simulink model "ADRC_Quanser"  (R2024a)
settings: Solver=ode1be  StartTime=0.0  StopTime=10  FixedStep=0.005  RelTol=1e-3
values from neighbouring files (symbols this model uses):
  dt = settings.dt    [Forward_Dynamics.m]    (also in Inverse_Dynamics.m; Settings.m = 0.005)
  l = settings.l    [Forward_Dynamics.m]    (also in Inverse_Dynamics.m; Settings.m = 0.127)
  omega_c = 1    [Inverse_Dynamics.m]    (also in Strojenie.m = 10^(omega_c_range(j)); Wykresy3D.m = 0.5*(omega_c_ISE + omega_c_IAE))
  P0 = [l;-l]    [Forward_Dynamics.m]    (also in Inverse_Dynamics.m)
  q0 = [0; -l/2; 3/2*pi; l/2; -l; 0; l; -l/2; pi/2; 3/2*l;0;0;-L; l;-l]    [Forward_Dynamics.m]    (also in Inverse_Dynamics.m)
libraries: slctrl_adaptive x6
settings Model: Creator=janek  LastModifiedBy=janek

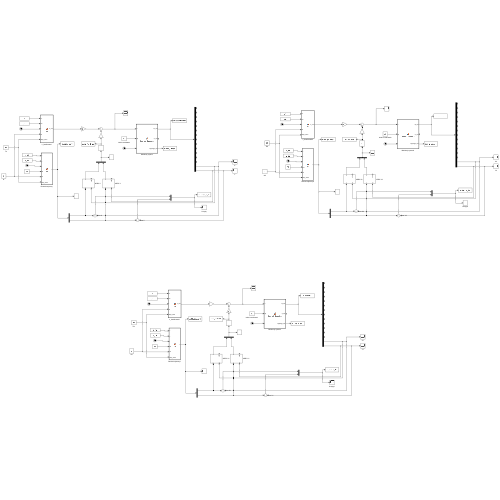
[thumbnail: Simulink's stored preview of the top-level diagram]
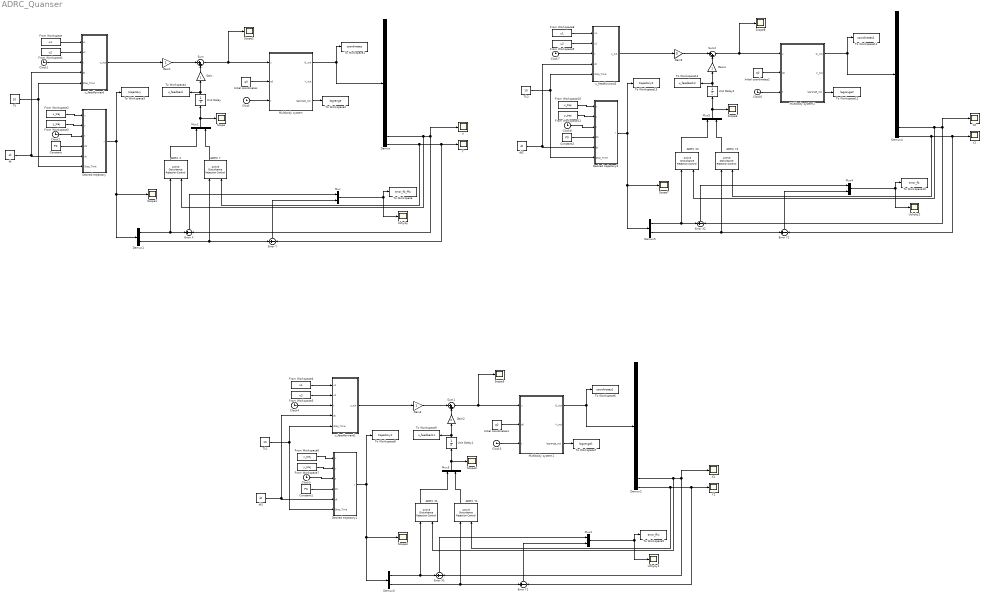
== system ADRC_Quanser ==
  ADRC X : slctrl_adaptive/Active Disturbance Rejection Control  time_domain=discrete-time  Ts=0.005  model_type=second-order  b0=b_hat  wc=omega_c*1  wo=omega_c*10  x0=[l;0;0]  ulim_checkbox=off  umax=inf  umin=-inf  xhat_checkbox=on
      settings: LibrarySourceBlock=slctrlblks/Adaptive Control/Active Disturbance Rejection Control
  ADRC X1 : slctrl_adaptive/Active Disturbance Rejection Control  time_domain=discrete-time  Ts=0.005  model_type=second-order  b0=b_hat  wc=omega_c*1  wo=omega_c*10  x0=[l;0;0]  ulim_checkbox=off  umax=inf  umin=-inf  xhat_checkbox=on
      settings: LibrarySourceBlock=slctrlblks/Adaptive Control/Active Disturbance Rejection Control
  ADRC X2 : slctrl_adaptive/Active Disturbance Rejection Control  time_domain=discrete-time  Ts=0.005  model_type=second-order  b0=b_hat  wc=omega_c*1  wo=omega_c*10  x0=[l;0;0]  ulim_checkbox=off  umax=inf  umin=-inf  xhat_checkbox=on
      settings: LibrarySourceBlock=slctrlblks/Adaptive Control/Active Disturbance Rejection Control
  ADRC Y : slctrl_adaptive/Active Disturbance Rejection Control  time_domain=discrete-time  Ts=0.005  model_type=second-order  b0=b_hat  wc=omega_c*1  wo=omega_c*10  x0=[-l;0;0]  ulim_checkbox=off  umax=inf  umin=-inf  xhat_checkbox=on
      settings: LibrarySourceBlock=slctrlblks/Adaptive Control/Active Disturbance Rejection Control
  ADRC Y1 : slctrl_adaptive/Active Disturbance Rejection Control  time_domain=discrete-time  Ts=0.005  model_type=second-order  b0=b_hat  wc=omega_c*1  wo=omega_c*10  x0=[-l;0;0]  ulim_checkbox=off  umax=inf  umin=-inf  xhat_checkbox=on
      settings: LibrarySourceBlock=slctrlblks/Adaptive Control/Active Disturbance Rejection Control
  ADRC Y2 : slctrl_adaptive/Active Disturbance Rejection Control  time_domain=discrete-time  Ts=0.005  model_type=second-order  b0=b_hat  wc=omega_c*1  wo=omega_c*10  x0=[-l;0;0]  ulim_checkbox=off  umax=inf  umin=-inf  xhat_checkbox=on
      settings: LibrarySourceBlock=slctrlblks/Adaptive Control/Active Disturbance Rejection Control
  Clock{,1..8} (9 alike) : Clock
  Constant : Constant  Value=P0
  Constant1 : Constant  Value=P0
  Constant2 : Constant  Value=P0
  Demux : Demux  Outputs=15
  Demux1 : Demux  Outputs=2
  Demux2 : Demux  Outputs=15
  Demux3 : Demux  Outputs=2
  Demux4 : Demux  Outputs=15
  Demux5 : Demux  Outputs=2
  Desired trajectory : MATLAB Function  TreatAsAtomicUnit=on
  Desired trajectory1 : MATLAB Function  TreatAsAtomicUnit=on
  Desired trajectory2 : MATLAB Function  TreatAsAtomicUnit=on
  Error X : Sum  Inputs=+|-
  Error X1 : Sum  Inputs=+|-
  Error X2 : Sum  Inputs=+|-
  Error Y : Sum  Inputs=+|-
  Error Y1 : Sum  Inputs=+|-
  Error Y2 : Sum  Inputs=+|-
  From Workspace : FromWorkspace  VariableName=u1  OutDataTypeStr=double  SampleTime=0.01
  From Workspace1 : FromWorkspace  VariableName=u2
  From Workspace10 : FromWorkspace  VariableName=x_traj
  From Workspace11 : FromWorkspace  VariableName=y_traj
  From Workspace2 : FromWorkspace  VariableName=x_traj
  From Workspace3 : FromWorkspace  VariableName=y_traj
  From Workspace4 : FromWorkspace  VariableName=u1  OutDataTypeStr=double  SampleTime=0.01
  From Workspace5 : FromWorkspace  VariableName=u2
  From Workspace6 : FromWorkspace  VariableName=x_traj
  From Workspace7 : FromWorkspace  VariableName=y_traj
  From Workspace8 : FromWorkspace  VariableName=u1  OutDataTypeStr=double  SampleTime=0.01
  From Workspace9 : FromWorkspace  VariableName=u2
  Gain{,1,3..4} (4 alike) : Gain
  Gain2 : Gain  Gain=0
  Gain5 : Gain  Gain=0
  Initial coordinates : Constant  Value=q0
  Initial coordinates1 : Constant  Value=q0
  Initial coordinates2 : Constant  Value=q0
  Multibody system : MATLAB Function  TreatAsAtomicUnit=on
  Multibody system1 : MATLAB Function  TreatAsAtomicUnit=on
  Multibody system2 : MATLAB Function  TreatAsAtomicUnit=on
  Mux{,1..5} (6 alike) : Mux  Inputs=2
  Scope{,1..8} (9 alike) : Scope
  Sum : Sum  Inputs=|++
  Sum1 : Sum  Inputs=|++
  Sum2 : Sum  Inputs=|++
  Tk : Constant  Value=10
  Tk1 : Constant  Value=10
  Tk2 : Constant  Value=10
  To Workspace : ToWorkspace  VariableName=error_fb_ffw  SaveFormat=Timeseries  SampleTime=-1
  To Workspace1 : ToWorkspace  VariableName=coordinates  SaveFormat=Timeseries  SampleTime=-1
  To Workspace10 : ToWorkspace  VariableName=error_fb  SaveFormat=Timeseries  SampleTime=-1
  To Workspace11 : ToWorkspace  VariableName=coordinates2  SaveFormat=Timeseries  SampleTime=-1
  To Workspace12 : ToWorkspace  VariableName=lagrange2  SaveFormat=Timeseries  SampleTime=-1
  To Workspace13 : ToWorkspace  VariableName=trajectory2  SaveFormat=Timeseries  SampleTime=-1
  To Workspace14 : ToWorkspace  VariableName=u_feedback2  SaveFormat=Timeseries  SampleTime=-1
  To Workspace2 : ToWorkspace  VariableName=lagrange  SaveFormat=Timeseries  SampleTime=-1
  To Workspace3 : ToWorkspace  VariableName=trajectory  SaveFormat=Timeseries  SampleTime=-1
  To Workspace4 : ToWorkspace  VariableName=u_feedback  SaveFormat=Timeseries  SampleTime=-1
  To Workspace5 : ToWorkspace  VariableName=error_ffw  SaveFormat=Timeseries  SampleTime=-1
  To Workspace6 : ToWorkspace  VariableName=coordinates1  SaveFormat=Timeseries  SampleTime=-1
  To Workspace7 : ToWorkspace  VariableName=lagrange1  SaveFormat=Timeseries  SampleTime=-1
  To Workspace8 : ToWorkspace  VariableName=trajectory1  SaveFormat=Timeseries  SampleTime=-1
  To Workspace9 : ToWorkspace  VariableName=u_feedback1  SaveFormat=Timeseries  SampleTime=-1
  Uchyby : Scope
  Uchyby1 : Scope
  Uchyby2 : Scope
  Unit Delay : UnitDelay  SampleTime=-1  HasFrameUpgradeWarning=on
  Unit Delay1 : UnitDelay  SampleTime=-1  HasFrameUpgradeWarning=on
  Unit Delay2 : UnitDelay  SampleTime=-1  HasFrameUpgradeWarning=on
  X : Scope
  X1 : Scope
  X2 : Scope
  Y : Scope
  Y1 : Scope
  Y2 : Scope
  dt : Constant  Value=dt
  dt1 : Constant  Value=dt
  dt2 : Constant  Value=dt
  u_feedforward : MATLAB Function  TreatAsAtomicUnit=on
  u_feedforward1 : MATLAB Function  TreatAsAtomicUnit=on
  u_feedforward2 : MATLAB Function  TreatAsAtomicUnit=on
  wires:
  Initial coordinates/1 -> Multibody system/2(q0)
  Multibody system/1(Q_out) -> Demux/1, To Workspace1/1
  Demux/15 -> Y/1, Error Y/2, ADRC Y/2
  Demux/14 -> ADRC X/2, X/1, Error X/2
  Multibody system/3(lagrange_out) -> To Workspace2/1
  Sum/1 -> Multibody system/1(u), Scope2/1
  Demux1/1 -> Error X/1, ADRC X/1
  Demux1/2 -> Error Y/1, ADRC Y/1
  Mux/1 -> Uchyby/1, To Workspace/1
  Clock1/1 -> u_feedforward/3(t)
  From Workspace/1 -> u_feedforward/1(u1)
  From Workspace1/1 -> u_feedforward/2(u2)
  From Workspace2/1 -> Desired trajectory/1(x)
  From Workspace3/1 -> Desired trajectory/2(y)
  Clock2/1 -> Desired trajectory/3(t)
  Desired trajectory/1(r) -> To Workspace3/1, Demux1/1, Scope1/1
  Constant/1 -> Desired trajectory/4(P0)
  Error Y/1 -> Mux/2
  Error X/1 -> Mux/1
  u_feedforward/1(u_out) -> Gain1/1
  Tk/1 -> u_feedforward/5(Stop_Time), Desired trajectory/6(Stop_Time)
  Mux1/1 -> Unit Delay/1, Scope/1
  ADRC X/1 -> Mux1/1
  ADRC Y/1 -> Mux1/2
  Unit Delay/1 -> To Workspace4/1, Gain/1
  Clock/1 -> Multibody system/3(t)
  Gain/1 -> Sum/2
  Gain1/1 -> Sum/1
  dt/1 -> u_feedforward/4(dt), Desired trajectory/5(dt)
  Constant1/1 -> Desired trajectory1/4(P0)
  Gain3/1 -> Sum1/1
  Multibody system1/3(lagrange_out) -> To Workspace7/1
  Unit Delay1/1 -> To Workspace9/1, Gain2/1
  ADRC Y1/1 -> Mux3/2
  ADRC X1/1 -> Mux3/1
  Mux3/1 -> Unit Delay1/1, Scope3/1
  Error Y1/1 -> Mux2/2
  Demux2/14 -> ADRC X1/2, X1/1, Error X1/2
  Clock5/1 -> Desired trajectory1/3(t)
  From Workspace6/1 -> Desired trajectory1/1(x)
  Demux3/1 -> Error X1/1, ADRC X1/1
  From Workspace4/1 -> u_feedforward1/1(u1)
  From Workspace7/1 -> Desired trajectory1/2(y)
  Tk1/1 -> u_feedforward1/5(Stop_Time), Desired trajectory1/6(Stop_Time)
  Clock4/1 -> u_feedforward1/3(t)
  From Workspace5/1 -> u_feedforward1/2(u2)
  Error X1/1 -> Mux2/1
  Gain2/1 -> Sum1/2
  Multibody system1/1(Q_out) -> Demux2/1, To Workspace6/1
  u_feedforward1/1(u_out) -> Gain3/1
  Clock3/1 -> Multibody system1/3(t)
  Initial coordinates1/1 -> Multibody system1/2(q0)
  dt1/1 -> u_feedforward1/4(dt), Desired trajectory1/5(dt)
  Demux2/15 -> Y1/1, Error Y1/2, ADRC Y1/2
  Mux2/1 -> Uchyby1/1, To Workspace5/1
  Demux3/2 -> Error Y1/1, ADRC Y1/1
  Sum1/1 -> Multibody system1/1(u), Scope5/1
  Desired trajectory1/1(r) -> To Workspace8/1, Demux3/1, Scope4/1
  Constant2/1 -> Desired trajectory2/4(P0)
  Gain5/1 -> Sum2/1
  Multibody system2/3(lagrange_out) -> To Workspace12/1
  Unit Delay2/1 -> To Workspace14/1, Gain4/1
  ADRC Y2/1 -> Mux5/2
  ADRC X2/1 -> Mux5/1
  Mux5/1 -> Unit Delay2/1, Scope6/1
  Error Y2/1 -> Mux4/2
  Demux4/14 -> ADRC X2/2, X2/1, Error X2/2
  Clock8/1 -> Desired trajectory2/3(t)
  From Workspace10/1 -> Desired trajectory2/1(x)
  Demux5/1 -> Error X2/1, ADRC X2/1
  From Workspace8/1 -> u_feedforward2/1(u1)
  From Workspace11/1 -> Desired trajectory2/2(y)
  Tk2/1 -> u_feedforward2/5(Stop_Time), Desired trajectory2/6(Stop_Time)
  Clock7/1 -> u_feedforward2/3(t)
  From Workspace9/1 -> u_feedforward2/2(u2)
  Error X2/1 -> Mux4/1
  Gain4/1 -> Sum2/2
  Multibody system2/1(Q_out) -> Demux4/1, To Workspace11/1
  u_feedforward2/1(u_out) -> Gain5/1
  Clock6/1 -> Multibody system2/3(t)
  Initial coordinates2/1 -> Multibody system2/2(q0)
  dt2/1 -> u_feedforward2/4(dt), Desired trajectory2/5(dt)
  Demux4/15 -> Y2/1, Error Y2/2, ADRC Y2/2
  Mux4/1 -> Uchyby2/1, To Workspace10/1
  Demux5/2 -> Error Y2/1, ADRC Y2/1
  Sum2/1 -> Multibody system2/1(u), Scope8/1
  Desired trajectory2/1(r) -> To Workspace13/1, Demux5/1, Scope7/1

== matlab function ADRC_Quanser/u_feedforward2 ==
  data: u1 input; u2 input; u_out output; t input; dt input; Stop_Time input
function u_out = fcn(u1, u2, t, dt,  Stop_Time)
if t == Stop_Time
    u_out = [0; 0];
else
u_out = [u1(round(t*1/dt) + 1); u2(round(t*1/dt) + 1)];
end

== matlab function ADRC_Quanser/Desired trajectory1 ==
  data: x input; r output; y input; t input; P0 input; dt input; Stop_Time input
function r = fcn(x, y, t,P0,dt, Stop_Time)
if t == Stop_Time   
    r = [P0(1);P0(2)];
else
    r = [x(round(t*1/dt)+1); y(round(1/dt*t)+1)];
end

== matlab function ADRC_Quanser/Desired trajectory ==
  data: x input; r output; y input; t input; P0 input; dt input; Stop_Time input
function r = fcn(x, y, t,P0,dt, Stop_Time)
if t == Stop_Time   
    r = [P0(1);P0(2)];
else
    r = [x(round(t*1/dt)+1); y(round(1/dt*t)+1)];
end

== matlab function ADRC_Quanser/Multibody system ==
  settings: updateMethod=DISCRETE
  data: u input; Q_out output; q0 input; V_out output; lagrange_out output; t input
function [Q_out, V_out, lagrange_out] = Forward_Dynamics(u, q0, t)
l = 0.127;
L = l*2;
m1 = 0.065;
m2 = 0.5*m1;
J = 9.5e-5;
g = 9.81;
M = 1.2*diag([m1,m1,J, m1,m1,J, m1,m1,J, m1,m1,J, m2,m2,m2]);

q0 = q0(1:13);
persistent initial_guess;

if isempty(initial_guess)
        % Initialize at first call
        initial_guess = [q0;l;-l; zeros(26,1)]; 
end


options = optimoptions('fsolve', 'Algorithm', 'levenberg-marquardt','FunctionTolerance', 1e-10);

func = @(unknowns)FD(unknowns, initial_guess(1:15),initial_guess(16:30),u,M,l,L,t);
solution = fsolve(func, initial_guess, options);
initial_guess = solution; % Update the guess for the next call

Q_out = solution(1:15);
V_out = solution(16:30);
lagrange_out = solution(31:end);


function solution = FD(unknowns, q, v, u, M, l, L, t)
Q = unknowns(1:15);
V = unknowns(16:30);
Lag = unknowns(31:end);

m2 = M(13,13);
g = 9.81;
dt = 0.005;



Wiatr = 0;
%WIATR
if t >= 3 && t <=3.5
    Wiatr = m2*g/100;
end

F = [0;0;u(1); 0;0;0; 0;0;0; 0;0;u(2); -m2*g;0;0];
C = Phiq(Q(1:13),Q(14:15),l);
wiezy = Phi(Q(1:13),Q(14:15),l,L);

alpha = 100;
beta = 100;

A = [M C'; C zeros(11,11)];
b = [F;Gamma(Q,V,l) - 2*alpha*C*V - beta^2*wiezy];
x = A\b;

a = x(1:15);
lagrange = x(16:end);

solution = [
V - (Q - q)/dt;
a - (V - v)/dt;
Lag - lagrange;
];

end

function jakobi = Phiq(q,p,l)
q3 = q(3);
q6 = q(6);
q9 = q(9);
q12 = q(12);
q13 = q(13);
p1 = p(1);
p2 = p(2);

jakobi=[
[-1,  0,                                                                                                                                                             -(l*sin(q3))/2,  0,  0,                                                                                                                                                                          0,  0,  0,              0,  0,  0,               0,                                                                                   0,                                                                                                                       0,                                                                                                                       0]
[ 0, -1,                                                                                                                                                              (l*cos(q3))/2,  0,  0,                                                                                                                                                                          0,  0,  0,              0,  0,  0,               0,                                                                                   0,                                                                                                                       0,                                                                                                                       0]
[ 0,  0,                                                                                                                                                                 -l*sin(q3), -1,  0,                                                                                                                                                             -(l*sin(q6))/2,  0,  0,              0,  0,  0,               0,                                                                                   0,                                                                                                                       0,                                                                                                                       0]
[ 0,  0,                                                                                                                                                                  l*cos(q3),  0, -1,                                                                                                                                                              (l*cos(q6))/2,  0,  0,              0,  0,  0,               0,                                                                                   0,                                                                                                                       0,                                                                                                                       0]
[ 0,  0,                                                                                                                                                                 -l*sin(q3),  0,  0,                                                                                                                                                                 -l*sin(q6), -1,  0, -(l*sin(q9))/2,  0,  0,               0,                                                                                   0,                                                                                                                       0,                                                                                                                       0]
[ 0,  0,                                                                                                                                                                  l*cos(q3),  0,  0,                                                                                                                                                                  l*cos(q6),  0, -1,  (l*cos(q9))/2,  0,  0,               0,                                                                                   0,                                                                                                                       0,                                                                                                                       0]
[ 0,  0,                                                                                                                                                                 -l*sin(q3),  0,  0,                                                                                                                                                                 -l*sin(q6),  0,  0,     -l*sin(q9), -1,  0, -(l*sin(q12))/2,                                                                                   0,                                                                                                                       0,                                                                                                                       0]
[ 0,  0,                                                                                                                                                                  l*cos(q3),  0,  0,                                                                                                                                                                  l*cos(q6),  0,  0,      l*cos(q9),  0, -1,  (l*cos(q12))/2,                                                                                   0,                                                                                                                       0,                                                                                                                       0]
[ 0,  0,                                                                                                                                                                 -l*sin(q3),  0,  0,                                                                                                                                                                 -l*sin(q6),  0,  0,     -l*sin(q9),  0,  0,     -l*sin(q12),                                                                                   0,                                                                                                                       0,                                                                                                                       0]
[ 0,  0,                                                                                                                                                                  l*cos(q3),  0,  0,                                                                                                                                                                  l*cos(q6),  0,  0,      l*cos(q9),  0,  0,      l*cos(q12),                                                                                   0,                                                                                                                       0,                                                                                                                       0]
[ 0,  0, -(2*l*sin(q3)*(l*cos(q3) - p1 + l*cos(q6)) - 2*l*cos(q3)*(l*sin(q3) - p2 + l*sin(q6)))/(2*((l*cos(q3) - p1 + l*cos(q6))^2 + q13^2 + (l*sin(q3) - p2 + l*sin(q6))^2)^(1/2)),  0,  0, -(2*l*sin(q6)*(l*cos(q3) - p1 + l*cos(q6)) - 2*l*cos(q6)*(l*sin(q3) - p2 + l*sin(q6)))/(2*((l*cos(q3) - p1 + l*cos(q6))^2 + q13^2 + (l*sin(q3) - p2 + l*sin(q6))^2)^(1/2)),  0,  0,              0,  0,  0,               0, q13/((l*cos(q3) - p1 + l*cos(q6))^2 + q13^2 + (l*sin(q3) - p2 + l*sin(q6))^2)^(1/2), -(2*l*cos(q3) - 2*p1 + 2*l*cos(q6))/(2*((l*cos(q3) - p1 + l*cos(q6))^2 + q13^2 + (l*sin(q3) - p2 + l*sin(q6))^2)^(1/2)), -(2*l*sin(q3) - 2*p2 + 2*l*sin(q6))/(2*((l*cos(q3) - p1 + l*cos(q6))^2 + q13^2 + (l*sin(q3) - p2 + l*sin(q6))^2)^(1/2))]
 
];
end

function wiezy = Phi(q,p,l,L)
q1 = q(1);
q2 = q(2);
q3 = q(3);
q4 = q(4);
q5 = q(5);
q6 = q(6);
q7 = q(7);
q8 = q(8);
q9 = q(9);
q10 = q(10);
q11 = q(11);
q12 = q(12);
q13 = q(13);
p1 = p(1);
p2 = p(2);

wiezy =[

 
                                                                 (l*cos(q3))/2 - q1;
                                                                 (l*sin(q3))/2 - q2;
                                                     l*cos(q3) - q4 + (l*cos(q6))/2;
                                                     l*sin(q3) - q5 + (l*sin(q6))/2;
                                         l*cos(q3) - q7 + l*cos(q6) + (l*cos(q9))/2;
                                         l*sin(q3) - q8 + l*sin(q6) + (l*sin(q9))/2;
                           l*cos(q3) - q10 + l*cos(q6) + l*cos(q9) + (l*cos(q12))/2;
                           l*sin(q3) - q11 + l*sin(q6) + l*sin(q9) + (l*sin(q12))/2;
                               l*cos(q3) - 2*l + l*cos(q6) + l*cos(q9) + l*cos(q12);
                                     l*sin(q3) + l*sin(q6) + l*sin(q9) + l*sin(q12);
((l*cos(q3) - p1 + l*cos(q6))^2 + q13^2 + (l*sin(q3) - p2 + l*sin(q6))^2)^(1/2) - L;
];
 
                                                                
end

end

== matlab function ADRC_Quanser/u_feedforward ==
  data: u1 input; u2 input; u_out output; t input; dt input; Stop_Time input
function u_out = fcn(u1, u2, t, dt,  Stop_Time)
if t == Stop_Time
    u_out = [0; 0];
else
u_out = [u1(round(t*1/dt) + 1); u2(round(t*1/dt) + 1)];
end

== matlab function ADRC_Quanser/Multibody system1 ==
  settings: updateMethod=DISCRETE
  data: u input; Q_out output; q0 input; V_out output; lagrange_out output; t input
function [Q_out, V_out, lagrange_out] = Forward_Dynamics(u, q0, t)
l = 0.127;
L = l*2;
m1 = 0.065;
m2 = 0.5*m1;
J = 9.5e-5;
g = 9.81;
M = 1.2*diag([m1,m1,J, m1,m1,J, m1,m1,J, m1,m1,J, m2,m2,m2]);

q0 = q0(1:13);
persistent initial_guess;

if isempty(initial_guess)
        % Initialize at first call
        initial_guess = [q0;l;-l; zeros(26,1)]; 
end


options = optimoptions('fsolve', 'Algorithm', 'levenberg-marquardt','FunctionTolerance', 1e-10);

func = @(unknowns)FD(unknowns, initial_guess(1:15),initial_guess(16:30),u,M,l,L,t);
solution = fsolve(func, initial_guess, options);
initial_guess = solution; % Update the guess for the next call

Q_out = solution(1:15);
V_out = solution(16:30);
lagrange_out = solution(31:end);


function solution = FD(unknowns, q, v, u, M, l, L, t)
Q = unknowns(1:15);
V = unknowns(16:30);
Lag = unknowns(31:end);

m2 = M(13,13);
g = 9.81;
dt = 0.005;



Wiatr = 0;
%WIATR
if t >= 3 && t <=3.5
    Wiatr = m2*g/100;
end

F = [0;0;u(1); 0;0;0; 0;0;0; 0;0;u(2); -m2*g;0;0];
C = Phiq(Q(1:13),Q(14:15),l);
wiezy = Phi(Q(1:13),Q(14:15),l,L);

alpha = 100;
beta = 100;

A = [M C'; C zeros(11,11)];
b = [F;Gamma(Q,V,l) - 2*alpha*C*V - beta^2*wiezy];
x = A\b;

a = x(1:15);
lagrange = x(16:end);

solution = [
V - (Q - q)/dt;
a - (V - v)/dt;
Lag - lagrange;
];

end

function jakobi = Phiq(q,p,l)
q3 = q(3);
q6 = q(6);
q9 = q(9);
q12 = q(12);
q13 = q(13);
p1 = p(1);
p2 = p(2);

jakobi=[
[-1,  0,                                                                                                                                                             -(l*sin(q3))/2,  0,  0,                                                                                                                                                                          0,  0,  0,              0,  0,  0,               0,                                                                                   0,                                                                                                                       0,                                                                                                                       0]
[ 0, -1,                                                                                                                                                              (l*cos(q3))/2,  0,  0,                                                                                                                                                                          0,  0,  0,              0,  0,  0,               0,                                                                                   0,                                                                                                                       0,                                                                                                                       0]
[ 0,  0,                                                                                                                                                                 -l*sin(q3), -1,  0,                                                                                                                                                             -(l*sin(q6))/2,  0,  0,              0,  0,  0,               0,                                                                                   0,                                                                                                                       0,                                                                                                                       0]
[ 0,  0,                                                                                                                                                                  l*cos(q3),  0, -1,                                                                                                                                                              (l*cos(q6))/2,  0,  0,              0,  0,  0,               0,                                                                                   0,                                                                                                                       0,                                                                                                                       0]
[ 0,  0,                                                                                                                                                                 -l*sin(q3),  0,  0,                                                                                                                                                                 -l*sin(q6), -1,  0, -(l*sin(q9))/2,  0,  0,               0,                                                                                   0,                                                                                                                       0,                                                                                                                       0]
[ 0,  0,                                                                                                                                                                  l*cos(q3),  0,  0,                                                                                                                                                                  l*cos(q6),  0, -1,  (l*cos(q9))/2,  0,  0,               0,                                                                                   0,                                                                                                                       0,                                                                                                                       0]
[ 0,  0,                                                                                                                                                                 -l*sin(q3),  0,  0,                                                                                                                                                                 -l*sin(q6),  0,  0,     -l*sin(q9), -1,  0, -(l*sin(q12))/2,                                                                                   0,                                                                                                                       0,                                                                                                                       0]
[ 0,  0,                                                                                                                                                                  l*cos(q3),  0,  0,                                                                                                                                                                  l*cos(q6),  0,  0,      l*cos(q9),  0, -1,  (l*cos(q12))/2,                                                                                   0,                                                                                                                       0,                                                                                                                       0]
[ 0,  0,                                                                                                                                                                 -l*sin(q3),  0,  0,                                                                                                                                                                 -l*sin(q6),  0,  0,     -l*sin(q9),  0,  0,     -l*sin(q12),                                                                                   0,                                                                                                                       0,                                                                                                                       0]
[ 0,  0,                                                                                                                                                                  l*cos(q3),  0,  0,                                                                                                                                                                  l*cos(q6),  0,  0,      l*cos(q9),  0,  0,      l*cos(q12),                                                                                   0,                                                                                                                       0,                                                                                                                       0]
[ 0,  0, -(2*l*sin(q3)*(l*cos(q3) - p1 + l*cos(q6)) - 2*l*cos(q3)*(l*sin(q3) - p2 + l*sin(q6)))/(2*((l*cos(q3) - p1 + l*cos(q6))^2 + q13^2 + (l*sin(q3) - p2 + l*sin(q6))^2)^(1/2)),  0,  0, -(2*l*sin(q6)*(l*cos(q3) - p1 + l*cos(q6)) - 2*l*cos(q6)*(l*sin(q3) - p2 + l*sin(q6)))/(2*((l*cos(q3) - p1 + l*cos(q6))^2 + q13^2 + (l*sin(q3) - p2 + l*sin(q6))^2)^(1/2)),  0,  0,              0,  0,  0,               0, q13/((l*cos(q3) - p1 + l*cos(q6))^2 + q13^2 + (l*sin(q3) - p2 + l*sin(q6))^2)^(1/2), -(2*l*cos(q3) - 2*p1 + 2*l*cos(q6))/(2*((l*cos(q3) - p1 + l*cos(q6))^2 + q13^2 + (l*sin(q3) - p2 + l*sin(q6))^2)^(1/2)), -(2*l*sin(q3) - 2*p2 + 2*l*sin(q6))/(2*((l*cos(q3) - p1 + l*cos(q6))^2 + q13^2 + (l*sin(q3) - p2 + l*sin(q6))^2)^(1/2))]
 
];
end

function wiezy = Phi(q,p,l,L)
q1 = q(1);
q2 = q(2);
q3 = q(3);
q4 = q(4);
q5 = q(5);
q6 = q(6);
q7 = q(7);
q8 = q(8);
q9 = q(9);
q10 = q(10);
q11 = q(11);
q12 = q(12);
q13 = q(13);
p1 = p(1);
p2 = p(2);

wiezy =[

 
                                                                 (l*cos(q3))/2 - q1;
                                                                 (l*sin(q3))/2 - q2;
                                                     l*cos(q3) - q4 + (l*cos(q6))/2;
                                                     l*sin(q3) - q5 + (l*sin(q6))/2;
                                         l*cos(q3) - q7 + l*cos(q6) + (l*cos(q9))/2;
                                         l*sin(q3) - q8 + l*sin(q6) + (l*sin(q9))/2;
                           l*cos(q3) - q10 + l*cos(q6) + l*cos(q9) + (l*cos(q12))/2;
                           l*sin(q3) - q11 + l*sin(q6) + l*sin(q9) + (l*sin(q12))/2;
                               l*cos(q3) - 2*l + l*cos(q6) + l*cos(q9) + l*cos(q12);
                                     l*sin(q3) + l*sin(q6) + l*sin(q9) + l*sin(q12);
((l*cos(q3) - p1 + l*cos(q6))^2 + q13^2 + (l*sin(q3) - p2 + l*sin(q6))^2)^(1/2) - L;
];
 
                                                                
end

end

== matlab function ADRC_Quanser/u_feedforward1 ==
  data: u1 input; u2 input; u_out output; t input; dt input; Stop_Time input
function u_out = fcn(u1, u2, t, dt,  Stop_Time)
if t == Stop_Time
    u_out = [0; 0];
else
u_out = [u1(round(t*1/dt) + 1); u2(round(t*1/dt) + 1)];
end

== matlab function ADRC_Quanser/Desired trajectory2 ==
  data: x input; r output; y input; t input; P0 input; dt input; Stop_Time input
function r = fcn(x, y, t,P0,dt, Stop_Time)
if t == Stop_Time   
    r = [P0(1);P0(2)];
else
    r = [x(round(t*1/dt)+1); y(round(1/dt*t)+1)];
end

== matlab function ADRC_Quanser/Multibody system2 ==
  settings: updateMethod=DISCRETE
  data: u input; Q_out output; q0 input; V_out output; lagrange_out output; t input
function [Q_out, V_out, lagrange_out] = Forward_Dynamics(u, q0, t)
l = 0.127;
L = l*2;
m1 = 0.065;
m2 = 0.5*m1;
J = 9.5e-5;
g = 9.81;
M = 1.2*diag([m1,m1,J, m1,m1,J, m1,m1,J, m1,m1,J, m2,m2,m2]);

q0 = q0(1:13);
persistent initial_guess;

if isempty(initial_guess)
        % Initialize at first call
        initial_guess = [q0;l;-l; zeros(26,1)]; 
end


options = optimoptions('fsolve', 'Algorithm', 'levenberg-marquardt','FunctionTolerance', 1e-10);

func = @(unknowns)FD(unknowns, initial_guess(1:15),initial_guess(16:30),u,M,l,L,t);
solution = fsolve(func, initial_guess, options);
initial_guess = solution; % Update the guess for the next call

Q_out = solution(1:15);
V_out = solution(16:30);
lagrange_out = solution(31:end);


function solution = FD(unknowns, q, v, u, M, l, L, t)
Q = unknowns(1:15);
V = unknowns(16:30);
Lag = unknowns(31:end);

m2 = M(13,13);
g = 9.81;
dt = 0.005;



Wiatr = 0;
%WIATR
if t >= 3 && t <=3.5
    Wiatr = m2*g/100;
end

F = [0;0;u(1); 0;0;0; 0;0;0; 0;0;u(2); -m2*g;0;0];
C = Phiq(Q(1:13),Q(14:15),l);
wiezy = Phi(Q(1:13),Q(14:15),l,L);

alpha = 100;
beta = 100;

A = [M C'; C zeros(11,11)];
b = [F;Gamma(Q,V,l) - 2*alpha*C*V - beta^2*wiezy];
x = A\b;

a = x(1:15);
lagrange = x(16:end);

solution = [
V - (Q - q)/dt;
a - (V - v)/dt;
Lag - lagrange;
];

end

function jakobi = Phiq(q,p,l)
q3 = q(3);
q6 = q(6);
q9 = q(9);
q12 = q(12);
q13 = q(13);
p1 = p(1);
p2 = p(2);

jakobi=[
[-1,  0,                                                                                                                                                             -(l*sin(q3))/2,  0,  0,                                                                                                                                                                          0,  0,  0,              0,  0,  0,               0,                                                                                   0,                                                                                                                       0,                                                                                                                       0]
[ 0, -1,                                                                                                                                                              (l*cos(q3))/2,  0,  0,                                                                                                                                                                          0,  0,  0,              0,  0,  0,               0,                                                                                   0,                                                                                                                       0,                                                                                                                       0]
[ 0,  0,                                                                                                                                                                 -l*sin(q3), -1,  0,                                                                                                                                                             -(l*sin(q6))/2,  0,  0,              0,  0,  0,               0,                                                                                   0,                                                                                                                       0,                                                                                                                       0]
[ 0,  0,                                                                                                                                                                  l*cos(q3),  0, -1,                                                                                                                                                              (l*cos(q6))/2,  0,  0,              0,  0,  0,               0,                                                                                   0,                                                                                                                       0,                                                                                                                       0]
[ 0,  0,                                                                                                                                                                 -l*sin(q3),  0,  0,                                                                                                                                                                 -l*sin(q6), -1,  0, -(l*sin(q9))/2,  0,  0,               0,                                                                                   0,                                                                                                                       0,                                                                                                                       0]
[ 0,  0,                                                                                                                                                                  l*cos(q3),  0,  0,                                                                                                                                                                  l*cos(q6),  0, -1,  (l*cos(q9))/2,  0,  0,               0,                                                                                   0,                                                                                                                       0,                                                                                                                       0]
[ 0,  0,                                                                                                                                                                 -l*sin(q3),  0,  0,                                                                                                                                                                 -l*sin(q6),  0,  0,     -l*sin(q9), -1,  0, -(l*sin(q12))/2,                                                                                   0,                                                                                                                       0,                                                                                                                       0]
[ 0,  0,                                                                                                                                                                  l*cos(q3),  0,  0,                                                                                                                                                                  l*cos(q6),  0,  0,      l*cos(q9),  0, -1,  (l*cos(q12))/2,                                                                                   0,                                                                                                                       0,                                                                                                                       0]
[ 0,  0,                                                                                                                                                                 -l*sin(q3),  0,  0,                                                                                                                                                                 -l*sin(q6),  0,  0,     -l*sin(q9),  0,  0,     -l*sin(q12),                                                                                   0,                                                                                                                       0,                                                                                                                       0]
[ 0,  0,                                                                                                                                                                  l*cos(q3),  0,  0,                                                                                                                                                                  l*cos(q6),  0,  0,      l*cos(q9),  0,  0,      l*cos(q12),                                                                                   0,                                                                                                                       0,                                                                                                                       0]
[ 0,  0, -(2*l*sin(q3)*(l*cos(q3) - p1 + l*cos(q6)) - 2*l*cos(q3)*(l*sin(q3) - p2 + l*sin(q6)))/(2*((l*cos(q3) - p1 + l*cos(q6))^2 + q13^2 + (l*sin(q3) - p2 + l*sin(q6))^2)^(1/2)),  0,  0, -(2*l*sin(q6)*(l*cos(q3) - p1 + l*cos(q6)) - 2*l*cos(q6)*(l*sin(q3) - p2 + l*sin(q6)))/(2*((l*cos(q3) - p1 + l*cos(q6))^2 + q13^2 + (l*sin(q3) - p2 + l*sin(q6))^2)^(1/2)),  0,  0,              0,  0,  0,               0, q13/((l*cos(q3) - p1 + l*cos(q6))^2 + q13^2 + (l*sin(q3) - p2 + l*sin(q6))^2)^(1/2), -(2*l*cos(q3) - 2*p1 + 2*l*cos(q6))/(2*((l*cos(q3) - p1 + l*cos(q6))^2 + q13^2 + (l*sin(q3) - p2 + l*sin(q6))^2)^(1/2)), -(2*l*sin(q3) - 2*p2 + 2*l*sin(q6))/(2*((l*cos(q3) - p1 + l*cos(q6))^2 + q13^2 + (l*sin(q3) - p2 + l*sin(q6))^2)^(1/2))]
 
];
end

function wiezy = Phi(q,p,l,L)
q1 = q(1);
q2 = q(2);
q3 = q(3);
q4 = q(4);
q5 = q(5);
q6 = q(6);
q7 = q(7);
q8 = q(8);
q9 = q(9);
q10 = q(10);
q11 = q(11);
q12 = q(12);
q13 = q(13);
p1 = p(1);
p2 = p(2);

wiezy =[

 
                                                                 (l*cos(q3))/2 - q1;
                                                                 (l*sin(q3))/2 - q2;
                                                     l*cos(q3) - q4 + (l*cos(q6))/2;
                                                     l*sin(q3) - q5 + (l*sin(q6))/2;
                                         l*cos(q3) - q7 + l*cos(q6) + (l*cos(q9))/2;
                                         l*sin(q3) - q8 + l*sin(q6) + (l*sin(q9))/2;
                           l*cos(q3) - q10 + l*cos(q6) + l*cos(q9) + (l*cos(q12))/2;
                           l*sin(q3) - q11 + l*sin(q6) + l*sin(q9) + (l*sin(q12))/2;
                               l*cos(q3) - 2*l + l*cos(q6) + l*cos(q9) + l*cos(q12);
                                     l*sin(q3) + l*sin(q6) + l*sin(q9) + l*sin(q12);
((l*cos(q3) - p1 + l*cos(q6))^2 + q13^2 + (l*sin(q3) - p2 + l*sin(q6))^2)^(1/2) - L;
];
 
                                                                
end

end
